simulink model "HTMPC_1"  (Simulink 9.1)
settings: Solver=ode45  StartTime=0.0  StopTime=6  FixedStep=0.01  RelTol=1e-3  EnableMultiTasking=on
libraries: simulink x5, Solver_SF x1
settings Model: Creator=xuwei  LastModifiedBy=CK12
settings DataIOCC: LimitDataPoints=on
settings OptimizationCC: ExpressionDepthLimit=2147483647
settings DebuggingCC: SolverPrmCheckMsg=warning  FcnCallInpInsideContextMsg=warning  StateNameClashWarn=warning
settings ConfigComp: CovHtmlReporting=off

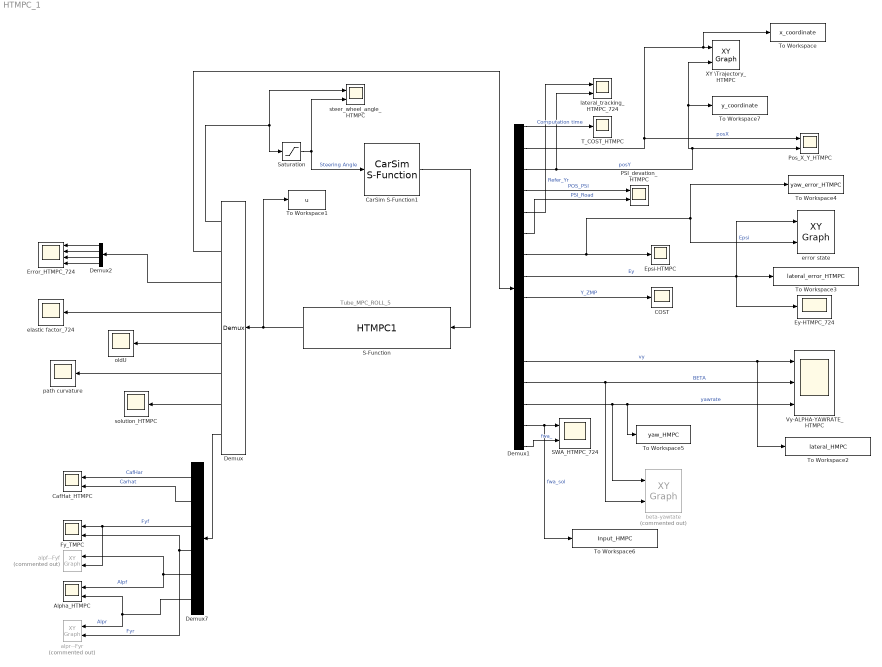
== system HTMPC_1 ==
  note: Tube_MPC_ROLL_5
  " Ey-HTMPC_724" : Scope
  Alpha_HTMPC : Scope  NumInputPorts=2
  COST : Scope
  CafHat_HTMPC : Scope  NumInputPorts=2
  CarSim S-Function1 : Solver_SF/CarSim S-Function  Priority=1  SIMFILE=simfile.sim  Run_RTs=off  vs_state_ind=Run  StopMode_ind=Vehicle Model
  Demux : Demux  Outputs=[1 16 4 5 5 5 1 6]
  Demux1 : Demux  Outputs=16
  Demux2 : Demux
  Demux7 : Demux  Outputs=6
  Epsi-HTMPC : Scope
  Error_HTMPC_724 : Scope  NumInputPorts=4
  Fy_TMPC : Scope  NumInputPorts=2
  PSI_devation_HTMPC : Scope  NumInputPorts=2
  Pos_X_Y_HTMPC : Scope  NumInputPorts=2
  S-Function : S-Function  FunctionName=HTMPC1  SFunctionDeploymentMode=off  EnableBusSupport=off
  SWA_HTMPC_724 : Scope  NumInputPorts=2
  Saturation : Saturate  UpperLimit=430  LowerLimit=-430
  T_COST_HTMPC : Scope
  To Workspace : ToWorkspace  VariableName=x_coordinate  SampleTime=-1
  To Workspace1 : ToWorkspace  VariableName=u  SaveFormat=Structure  SampleTime=-1
  To Workspace2 : ToWorkspace  VariableName=lateral_HMPC  SaveFormat=Timeseries  SampleTime=-1
  To Workspace3 : ToWorkspace  VariableName=lateral_error_HTMPC  SampleTime=-1
      settings: MaxDataPoints=120
  To Workspace4 : ToWorkspace  VariableName=yaw_error_HTMPC  SaveFormat=Timeseries  SampleTime=-1
  To Workspace5 : ToWorkspace  VariableName=yaw_HMPC  SaveFormat=Timeseries  SampleTime=-1
  To Workspace6 : ToWorkspace  VariableName=Input_HMPC  SampleTime=-1
  To Workspace7 : ToWorkspace  VariableName=y_coordinate  SampleTime=-1
  Vy-ALPHA-YAWRATE_HTMPC : Scope  NumInputPorts=3
  XY \Trajectory_HTMPC : simulink/Sinks/XY Graph  xmin=30  xmax=200  ymin=-0.5  ymax=4  st=-1
  alpf--Fyf : simulink/Sinks/XY Graph  Commented=on  xmin=-0.5  xmax=0.5  ymin=-10000  ymax=10000  st=-1
  alpr--Fyr : simulink/Sinks/XY Graph  Commented=on  xmin=-0.5  xmax=0.5  ymin=-8000  ymax=8000  st=-1
  beta-yawtate : simulink/Sinks/XY Graph  Commented=on  xmin=-0.7  xmax=0.7  ymin=-0.1  ymax=0.1  st=-1
  elastic factor_724 : Scope
  error state : simulink/Sinks/XY Graph  xmin=-0.1  xmax=0.1  ymin=-0.05  ymax=0.05  st=-1
  lateral_tracking_HTMPC_724 : Scope  NumInputPorts=2
  "oldU " : Scope
  path curvature : Scope
  "solution_HTMPC " : Scope
  steer_wheel_angle_HTMPC : Scope  NumInputPorts=2
  wires:
  CarSim S-Function1/1 -> S-Function/1
  S-Function/1 -> To Workspace1/1, Demux/1
  Demux/1 -> steer_wheel_angle_HTMPC/1, Saturation/1
  Demux/2 -> Demux1/1
  Demux2/1 -> Error_HTMPC_724/1
  Demux2/2 -> Error_HTMPC_724/2
  Demux2/3 -> Error_HTMPC_724/3
  Demux2/4 -> Error_HTMPC_724/4
  Demux/3 -> Demux2/1
  Demux1/8 -> To Workspace3/1, error state/1, " Ey-HTMPC_724"/1  "Ey"
  Demux1/2 -> To Workspace/1, XY \Trajectory_HTMPC/1, Pos_X_Y_HTMPC/1  "posX"
  Demux1/6 -> PSI_devation_HTMPC/2  "PSI_Road"
  Demux1/1 -> T_COST_HTMPC/1  "Computation time"
  Demux1/14 -> beta-yawtate/1, Vy-ALPHA-YAWRATE_HTMPC/3, To Workspace5/1  "yawrate"
  Demux1/4 -> PSI_devation_HTMPC/1  "POS_PSI"
  Demux1/3 -> To Workspace7/1, XY \Trajectory_HTMPC/2, Pos_X_Y_HTMPC/2, lateral_tracking_HTMPC_724/2  "posY"
  Demux1/7 -> error state/2, To Workspace4/1, Epsi-HTMPC/1  "Epsi"
  Demux1/9 -> COST/1  "Y_ZMP"
  Demux1/12 -> Vy-ALPHA-YAWRATE_HTMPC/1, To Workspace2/1  "vy"
  Demux1/5 -> lateral_tracking_HTMPC_724/1  "Refer_Yr"
  Demux1/13 -> Vy-ALPHA-YAWRATE_HTMPC/2, beta-yawtate/2  "BETA"
  Demux1/15 -> To Workspace6/1, SWA_HTMPC_724/1  "fwa_sol"
  Demux1/16 -> SWA_HTMPC_724/2  "fwa_"
  Demux/8 -> Demux7/1
  Demux7/1 -> CafHat_HTMPC/1  "CafHar"
  Demux7/2 -> CafHat_HTMPC/2  "Carhat"
  Demux7/3 -> Fy_TMPC/1, alpf--Fyf/2  "Fyf"
  Demux7/4 -> Fy_TMPC/2, alpr--Fyr/2  "Fyr"
  Demux7/5 -> alpf--Fyf/1, Alpha_HTMPC/1  "Alpf"
  Demux7/6 -> alpr--Fyr/1, Alpha_HTMPC/2  "Alpr"
  Saturation/1 -> steer_wheel_angle_HTMPC/2, CarSim S-Function1/1  "Steering Angle"
  Demux/7 -> "solution_HTMPC "/1
  Demux/6 -> path curvature/1
  Demux/4 -> elastic factor_724/1
  Demux/5 -> "oldU "/1
